simulink model "OMAP"  (R2018b)
settings: Solver=FixedStepDiscrete  StartTime=0.0  StopTime=10.0  FixedStep=0.01  RelTol=1e-3
values from neighbouring files (symbols this model uses):
  Clb_ICADirect_LaneDisp_StateFive = Simulink.Parameter    [omap_ver_442.m]
  Clb_ICADirect_LaneDisp_StateFour = Simulink.Parameter    [omap_ver_442.m]
  Clb_ICADirect_LaneDisp_StateOne = Simulink.Parameter    [omap_ver_442.m]
  Clb_ICADirect_LaneDisp_StateThree = Simulink.Parameter    [omap_ver_442.m]
  Clb_ICADirect_LaneDisp_StateTwo = Simulink.Parameter    [omap_ver_442.m]
  Clb_ICADirect_LaneDisp_StateZero = Simulink.Parameter    [omap_ver_442.m]
  Clb_ICADirect_LaneDispSW = Simulink.Parameter    [omap_ver_442.m]
  Clb_ICADirect_TrnLghtsCom_Switch = Simulink.Parameter    [omap_ver_442.m]
  Clb_ICADirect_TrnLghtsCom_Value = Simulink.Parameter    [omap_ver_442.m]
  Clb_ICADirect_TrnLghtsCrtl_Inhb = Simulink.Parameter    [omap_ver_442.m]
  OMAP_ACCAEB_EMSESC_Decel = Simulink.Parameter    [omap_ver_442.m]
  OMAP_ACCFCW_IC_Decel = Simulink.Parameter    [omap_ver_442.m]
  OMAP_clb_ACC_RVVReqType = Simulink.Parameter    [omap_ver_442.m]
  OMAP_clb_ACC_RVVReqType_Switch = Simulink.Parameter    [omap_ver_442.m]
  OMAP_clb_ACCHeadwayDisplay = Simulink.Parameter    [omap_ver_442.m]
  OMAP_clb_ACCHeadwayDisplay_Switch = Simulink.Parameter    [omap_ver_442.m]
  OMAP_clb_ACCHeadwayIcon = Simulink.Parameter    [omap_ver_442.m]
  OMAP_clb_ACCHeadwayIcon_Switch = Simulink.Parameter    [omap_ver_442.m]
  OMAP_clb_ACCMessagePrompt = Simulink.Parameter    [omap_ver_442.m]
  OMAP_clb_ACCMessagePrompt_Switch = Simulink.Parameter    [omap_ver_442.m]
  OMAP_clb_ACCRequestEPB = Simulink.Parameter    [omap_ver_442.m]
  OMAP_clb_ACCRequestEPB_Switch = Simulink.Parameter    [omap_ver_442.m]
  OMAP_clb_ACCSetSpeed = Simulink.Parameter    [omap_ver_442.m]
  OMAP_clb_ACCSetSpeed_Switch = Simulink.Parameter    [omap_ver_442.m]
  OMAP_clb_ACCSetSpeedDis = Simulink.Parameter    [omap_ver_442.m]
  OMAP_clb_ACCSetSpeedDis_Switch = Simulink.Parameter    [omap_ver_442.m]
  OMAP_clb_ACCState = Simulink.Parameter    [omap_ver_442.m]
  OMAP_clb_ACCState_Switch = Simulink.Parameter    [omap_ver_442.m]
  OMAP_clb_ACCStatusIconDis = Simulink.Parameter    [omap_ver_442.m]
  OMAP_clb_ACCStatusIconDis_Switch = Simulink.Parameter    [omap_ver_442.m]
  OMAP_clb_ACCTorqueReq = Simulink.Parameter    [omap_ver_442.m]
  OMAP_clb_ACCTorqueReq_Switch = Simulink.Parameter    [omap_ver_442.m]
  OMAP_clb_ADAS_State = Simulink.Parameter    [omap_ver_442.m]
  OMAP_clb_ADAS_State_Switch = Simulink.Parameter    [omap_ver_442.m]
  OMAP_clb_AEBAlertReq = Simulink.Parameter    [omap_ver_442.m]
  OMAP_clb_AEBAlertReq_Switch = Simulink.Parameter    [omap_ver_442.m]
  OMAP_clb_AEBBrakingProg = Simulink.Parameter    [omap_ver_442.m]
  OMAP_clb_AEBBrakingProg_Switch = Simulink.Parameter    [omap_ver_442.m]
  OMAP_clb_AEBFaultStatus = Simulink.Parameter    [omap_ver_442.m]
  OMAP_clb_AEBFaultStatus_Switch = Simulink.Parameter    [omap_ver_442.m]
  OMAP_clb_AEBMassageDisp = Simulink.Parameter    [omap_ver_442.m]
  OMAP_clb_AEBMassageDisp_Switch = Simulink.Parameter    [omap_ver_442.m]
  OMAP_clb_AEBState = Simulink.Parameter    [omap_ver_442.m]
  OMAP_clb_AEBState_Switch = Simulink.Parameter    [omap_ver_442.m]
  OMAP_clb_AEBSwitchStatus = Simulink.Parameter    [omap_ver_442.m]
  OMAP_clb_AEBSwitchStatus_Switch = Simulink.Parameter    [omap_ver_442.m]
  OMAP_clb_BrakeRequest = Simulink.Parameter    [omap_ver_442.m]
  OMAP_clb_BrakeRequest_Switch = Simulink.Parameter    [omap_ver_442.m]
  OMAP_clb_DecelerationSet = Simulink.Parameter    [omap_ver_442.m]
  OMAP_clb_DecelerationSet_Switch = Simulink.Parameter    [omap_ver_442.m]
  OMAP_clb_DecelerationType = Simulink.Parameter    [omap_ver_442.m]
  OMAP_clb_DecelerationType_Switch = Simulink.Parameter    [omap_ver_442.m]
  OMAP_clb_DeclControlReq = Simulink.Parameter    [omap_ver_442.m]
  OMAP_clb_DeclControlReq_Switch = Simulink.Parameter    [omap_ver_442.m]
  OMAP_clb_DownorUpGearMinTime = Simulink.Parameter    [omap_ver_442.m]
  OMAP_clb_DownorUpGearMinTime_Switch = Simulink.Parameter    [omap_ver_442.m]
  OMAP_clb_ELKPopupMessage = Simulink.Parameter    [omap_ver_442.m]
  OMAP_clb_ELKPopupMessage_Switch = Simulink.Parameter    [omap_ver_442.m]
  OMAP_clb_ELKSts = Simulink.Parameter    [omap_ver_442.m]
  OMAP_clb_ELKSts_Switch = Simulink.Parameter    [omap_ver_442.m]
  OMAP_clb_ESAFaultSt = Simulink.Parameter    [omap_ver_442.m]
  OMAP_clb_ESAFaultSt_Switch = Simulink.Parameter    [omap_ver_442.m]
  OMAP_clb_ESARequest = Simulink.Parameter    [omap_ver_442.m]
  OMAP_clb_ESARequest_Switch = Simulink.Parameter    [omap_ver_442.m]
  OMAP_clb_ESAState = Simulink.Parameter    [omap_ver_442.m]
  OMAP_clb_ESAState_Switch = Simulink.Parameter    [omap_ver_442.m]
  OMAP_clb_ESATorqueReq = Simulink.Parameter    [omap_ver_442.m]
  OMAP_clb_ESATorqueReq_Switch = Simulink.Parameter    [omap_ver_442.m]
  OMAP_clb_ESCDriveOff = Simulink.Parameter    [omap_ver_442.m]
  OMAP_clb_ESCDriveOff_Switch = Simulink.Parameter    [omap_ver_442.m]
  OMAP_clb_ESCHoldReq = Simulink.Parameter    [omap_ver_442.m]
  OMAP_clb_ESCHoldReq_Switch = Simulink.Parameter    [omap_ver_442.m]
  OMAP_clb_Handsoffwarning = Simulink.Parameter    [omap_ver_442.m]
  OMAP_clb_Handsoffwarning_Switch = Simulink.Parameter    [omap_ver_442.m]
  OMAP_clb_HapticAlarmReq = Simulink.Parameter    [omap_ver_442.m]
  OMAP_clb_HapticAlarmReq_Switch = Simulink.Parameter    [omap_ver_442.m]
  OMAP_clb_HMIPopupMassage = Simulink.Parameter    [omap_ver_442.m]
  OMAP_clb_HMIPopupMassage_Switch = Simulink.Parameter    [omap_ver_442.m]
  OMAP_clb_HWAActionSts = Simulink.Parameter    [omap_ver_442.m]
  OMAP_clb_HWAActionSts_Switch = Simulink.Parameter    [omap_ver_442.m]
  OMAP_clb_HWAMode = Simulink.Parameter    [omap_ver_442.m]
  OMAP_clb_HWAMode_Switch = Simulink.Parameter    [omap_ver_442.m]
  OMAP_clb_HWATurnOnIdctr = Simulink.Parameter    [omap_ver_442.m]
  OMAP_clb_HWATurnOnIdctr_Switch = Simulink.Parameter    [omap_ver_442.m]
  OMAP_clb_ICAMassageDisp = Simulink.Parameter    [omap_ver_442.m]
  OMAP_clb_ICAMassageDisp_Switch = Simulink.Parameter    [omap_ver_442.m]
  OMAP_clb_ICAStatusIcon = Simulink.Parameter    [omap_ver_442.m]
  OMAP_clb_ICAStatusIcon_Switch = Simulink.Parameter    [omap_ver_442.m]
  OMAP_clb_ISLCDriverRemind = Simulink.Parameter    [omap_ver_442.m]
  OMAP_clb_ISLCDriverRemind_Switch = Simulink.Parameter    [omap_ver_442.m]
  OMAP_clb_ISLCState = Simulink.Parameter    [omap_ver_442.m]
  OMAP_clb_ISLCState_Switch = Simulink.Parameter    [omap_ver_442.m]
  OMAP_clb_JAFaultSt = Simulink.Parameter    [omap_ver_442.m]
  OMAP_clb_JAFaultSt_Switch = Simulink.Parameter    [omap_ver_442.m]
  OMAP_clb_LCAPopupMessage = Simulink.Parameter    [omap_ver_442.m]
  OMAP_clb_LCAPopupMessage_Switch = Simulink.Parameter    [omap_ver_442.m]
  OMAP_clb_LCAStatusDisplay = Simulink.Parameter    [omap_ver_442.m]
  OMAP_clb_LCAStatusDisplay_Switch = Simulink.Parameter    [omap_ver_442.m]
  OMAP_clb_LDWStatusDisplay = Simulink.Parameter    [omap_ver_442.m]
  OMAP_clb_LDWStatusDisplay_Switch = Simulink.Parameter    [omap_ver_442.m]
  OMAP_clb_LDWWarningSt = Simulink.Parameter    [omap_ver_442.m]
  OMAP_clb_LDWWarningSt_Switch = Simulink.Parameter    [omap_ver_442.m]
  OMAP_clb_LightControlValid = Simulink.Parameter    [omap_ver_442.m]
  OMAP_clb_LightControlValid_Switch = Simulink.Parameter    [omap_ver_442.m]
  OMAP_clb_LKAActivation = Simulink.Parameter    [omap_ver_442.m]
  OMAP_clb_LKAActivation_Switch = Simulink.Parameter    [omap_ver_442.m]
  OMAP_clb_LKAAngleReq = Simulink.Parameter    [omap_ver_442.m]
  OMAP_clb_LKAAngleReq_Switch = Simulink.Parameter    [omap_ver_442.m]
  OMAP_clb_LKAMode = Simulink.Parameter    [omap_ver_442.m]
  OMAP_clb_LKAMode_Switch = Simulink.Parameter    [omap_ver_442.m]
  OMAP_clb_LKAorELK_CoolTime = Simulink.Parameter    [omap_ver_442.m]
  OMAP_clb_LKAState = Simulink.Parameter    [omap_ver_442.m]
  OMAP_clb_LKAState_Switch = Simulink.Parameter    [omap_ver_442.m]
  OMAP_clb_LKAStatusDisplay = Simulink.Parameter    [omap_ver_442.m]
  OMAP_clb_LKAStatusDisplay_Switch = Simulink.Parameter    [omap_ver_442.m]
  OMAP_clb_LKASwitchState = Simulink.Parameter    [omap_ver_442.m]
  OMAP_clb_LKASwitchState_Switch = Simulink.Parameter    [omap_ver_442.m]
  OMAP_clb_LKATorqFactReq = Simulink.Parameter    [omap_ver_442.m]
  OMAP_clb_LKATorqFactReq_Switch = Simulink.Parameter    [omap_ver_442.m]
  OMAP_clb_PrefillRequest = Simulink.Parameter    [omap_ver_442.m]
  ... (+36 more)
libraries: simulink x184, canmsglib x2
(part 1 of 14)
settings Model: Creator=许阁  LastModifiedBy=许阁
settings OptimizationCC: BlockReduction=off  DefaultParameterBehavior=Inlined  DefaultUnderspecifiedDataType=single  EnhancedBackFolding=on  PassReuseOutputArgsAs=Individual arguments  ZeroExternalMemoryAtStartup=off  ZeroInternalMemoryAtStartup=off  OptimizeBlockOrder=speed  DifferentSizesBufferReuse=on  OptimizationCustomize=off
settings DebuggingCC: ParameterTunabilityLossMsg=error
settings SFSimCC: MATLABDynamicMemAlloc=off
settings RTWCC: SystemTargetFile=autosar.tlc  GenCodeOnly=on  TemplateMakefile=ert_default_tmf  Description=AUTOSAR  GenerateReport=on  IncludeHyperlinkInReport=on  LaunchReport=on  GenerateTraceInfo=on  GenerateTraceReport=on  GenerateTraceReportSl=on  GenerateTraceReportSf=on  GenerateTraceReportEml=on  GenerateCodeMetricsReport=on
settings CodeAppCC: ForceParamTrailComments=on  IgnoreCustomStorageClasses=off  OperatorAnnotations=on  SimulinkDataObjDesc=on  SFDataObjDesc=on  InsertBlockDesc=on
settings STFCustomTargetCC: TargetLangStandard=C99 (ISO)  MultiwordLength=256  ParMdlRefBuildCompliant=on  CompOptLevelCompliant=on  IncludeMdlTerminateFcn=off  CombineOutputUpdateFcns=on  SuppressErrorStatus=on  ERTCustomFileBanners=on  SupportNonFinite=off  SupportComplex=off  SupportContinuousTime=off  SupportNonInlinedSFcns=off  RemoveResetFunc=on  MATLABClassNameForMDSCustomization=Simulink.SoftwareTarget.ERTCustomization  AutosarCompliant=on  UseToolchainInfoCompliant=on  LookupTableObjectStructAxisOrder=2,1,3,4,...  LUTObjectStructOrderEvenSpacing=Size,Table,Breakpoints  SystemTargetFile=autosar.tlc
settings ERTTargetCC: TargetLangStandard=C99 (ISO)  ConcurrentExecutionCompliant=off  IncludeMdlTerminateFcn=off  SuppressErrorStatus=on  SupportNonFinite=off  SupportComplex=off  ModelStepFunctionPrototypeControlCompliant=off  CPPClassGenCompliant=off  AutosarCompliant=on  LookupTableObjectStructAxisOrder=2,1,3,4,...  LUTObjectStructOrderEvenSpacing=Size,Table,Breakpoints  GenerateASAP2=on  InlinedParameterPlacement=NonHierarchical  ERTCustomFileTemplate=example_file_process.tlc

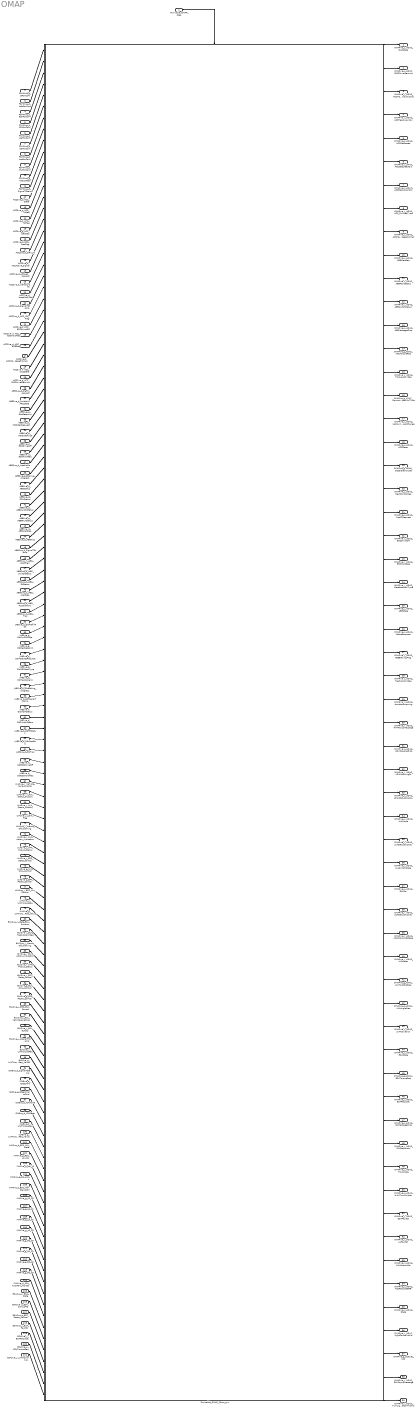
== system OMAP ==
  Runnable_OMAP_Step : Inport  SampleTime=0.01  OutputFunctionCall=on
  FDMMve_d_JaFcnConf : Inport  Port=2  OutDataTypeStr=UInt16  PortDimensions=1
  FDMMve_d_AebFcnConf : Inport  Port=3  OutDataTypeStr=UInt16  PortDimensions=1
  FDMMve_d_EsaFcnConf : Inport  Port=4  OutDataTypeStr=UInt16  PortDimensions=1
  FDMMve_d_ElkFcnConf : Inport  Port=5  OutDataTypeStr=UInt16  PortDimensions=1
  FDMMve_d_LkaFcnConf : Inport  Port=6  OutDataTypeStr=UInt16  PortDimensions=1
  FDMMve_d_IcaFcnConf : Inport  Port=7  OutDataTypeStr=UInt16  PortDimensions=1
  FDMMve_d_AccFcnConf : Inport  Port=8  OutDataTypeStr=UInt16  PortDimensions=1
  FDMMve_d_EwFcnConf : Inport  Port=9  OutDataTypeStr=UInt16  PortDimensions=1
  FDMMve_g_Adas2Fapa : Inport  Port=10  OutDataTypeStr=UInt32  PortDimensions=1
  FDMMve_d_SignalTStamp : Inport  Port=11  OutDataTypeStr=UInt16  PortDimensions=1
  ACCSve_d_ACC_State : Inport  Port=12  OutDataTypeStr=UInt16  PortDimensions=1
  ACCSve_g_ACC_TqReq : Inport  Port=13  OutDataTypeStr=T_M_Nm_Float32  PortDimensions=1
  ACCSve_d_ACC_TqFlag : Inport  Port=14  OutDataTypeStr=UInt16  PortDimensions=1
  ACCSve_g_ACC_DecReq : Inport  Port=15  OutDataTypeStr=T_M_Nm_Float32  PortDimensions=1
  ACCSve_d_ACC_DecFlag : Inport  Port=16  OutDataTypeStr=UInt16  PortDimensions=1
  ACCSve_d_CIPV_ID : Inport  Port=17  OutDataTypeStr=UInt16  PortDimensions=1
  ACCSve_d_ACCActive_Signal : Inport  Port=18  OutDataTypeStr=UInt16  PortDimensions=1
  ACCSve_d_ACC_go_request : Inport  Port=19  OutDataTypeStr=UInt16  PortDimensions=1
  ACCSve_d_VelocitySet : Inport  Port=20  OutDataTypeStr=UInt16  PortDimensions=1
  ACCSve_d_HeadWaySet : Inport  Port=21  OutDataTypeStr=UInt16  PortDimensions=1
  ACCSve_d_SignalTStamp : Inport  Port=22  OutDataTypeStr=UInt16  PortDimensions=1
  ACCSve_d_ACC_ICA_Flag : Inport  Port=23  OutDataTypeStr=UInt16  PortDimensions=1
  ACCSve_d_ACC_ESCDriveOff : Inport  Port=24  OutDataTypeStr=UInt16  PortDimensions=1
  ACCSve_d_ACC_ESCHoldReq : Inport  Port=25  OutDataTypeStr=UInt16  PortDimensions=1
  ACCSve_d_ACC_EPBReq : Inport  Port=26  OutDataTypeStr=UInt16  PortDimensions=1
  ACCSve_d_ACCMessagePrompt : Inport  Port=27  OutDataTypeStr=UInt16
  ACCSve_d_ACC_ISLCState : Inport  Port=28  OutDataTypeStr=UInt16  PortDimensions=1
  ACCSve_d_ACC_ISLCDriverRemind : Inport  Port=29  OutDataTypeStr=UInt16  PortDimensions=1
  AEBSve_d_Prefill_request : Inport  Port=30  OutDataTypeStr=UInt16  PortDimensions=1
  AEBSve_d_functionFARCState : Inport  Port=31  OutDataTypeStr=UInt16  PortDimensions=1
  AEBSve_g_DecSetpoint : Inport  Port=32  OutDataTypeStr=T_M_Nm_Float32  PortDimensions=1
  AEBSve_d_MDDdecRequest : Inport  Port=33  OutDataTypeStr=UInt16  PortDimensions=1
  AEBSve_d_MDDdecType : Inport  Port=34  OutDataTypeStr=UInt16  PortDimensions=1
  AEBSve_d_ESCDriveOff : Inport  Port=35  OutDataTypeStr=UInt16  PortDimensions=1
  AEBSve_d_ESCHoldReq : Inport  Port=36  OutDataTypeStr=UInt16  PortDimensions=1
  AEBSve_d_HapticAlarm : Inport  Port=37  OutDataTypeStr=UInt16  PortDimensions=1
  AEBSve_d_Braking_progress : Inport  Port=38  OutDataTypeStr=UInt16  PortDimensions=1
  AEBSve_d_AEBStatus : Inport  Port=39  OutDataTypeStr=UInt16  PortDimensions=1
  AEBSve_d_FCWStatus : Inport  Port=40  OutDataTypeStr=UInt16  PortDimensions=1
  AEBSve_d_AEBSwitchStatus : Inport  Port=41  OutDataTypeStr=UInt16  PortDimensions=1
  AEBSve_d_AEBFaultStatus : Inport  Port=42  OutDataTypeStr=UInt16  PortDimensions=1
  AEBSve_d_AEBAlertReq : Inport  Port=43  OutDataTypeStr=UInt16  PortDimensions=1
  AEBSve_d_AEBTips : Inport  Port=44  OutDataTypeStr=UInt16  PortDimensions=1
  AEBSve_d_SignalTStamp : Inport  Port=45  OutDataTypeStr=UInt16  PortDimensions=1
  AEBSve_d_JABS_AlertSign : Inport  Port=46  OutDataTypeStr=UInt16  PortDimensions=1
  AEBSve_d_JABS_SwitchStatus : Inport  Port=47  OutDataTypeStr=UInt16  PortDimensions=1
  AEBSve_d_JABS_FltStatus : Inport  Port=48  OutDataTypeStr=UInt16  PortDimensions=1
  AEBSve_d_JABS_AlertReq : Inport  Port=49  OutDataTypeStr=UInt16  PortDimensions=1
  AEBSve_d_JABS_HapticAlarm : Inport  Port=50  OutDataTypeStr=UInt16  PortDimensions=1
  AEBSve_d_JABS_Tips : Inport  Port=51  OutDataTypeStr=UInt16  PortDimensions=1
  JABSve_d_DbPrefillReq : Inport  Port=52  OutDataTypeStr=UInt16  PortDimensions=1
  JABSve_d_DbFunFARCSta : Inport  Port=53  OutDataTypeStr=UInt16  PortDimensions=1
  JABSve_g_DbDecSetpoint : Inport  Port=54  OutDataTypeStr=T_M_Nm_Float32  PortDimensions=1
  JABSve_d_DbMDDdecRequest : Inport  Port=55  OutDataTypeStr=UInt16  PortDimensions=1
  JABSve_d_DbMDDdecType : Inport  Port=56  OutDataTypeStr=UInt16  PortDimensions=1
  JABSve_d_DbHapticAlarm : Inport  Port=57  OutDataTypeStr=UInt16  PortDimensions=1
  JABSve_d_DbBraking_progress : Inport  Port=58  OutDataTypeStr=UInt16  PortDimensions=1
  JABSve_d_DbSignalTStamp : Inport  Port=59  OutDataTypeStr=UInt16  PortDimensions=1
  JABSve_d_DbJACWStatus : Inport  Port=60  OutDataTypeStr=UInt16  PortDimensions=1
  JABSve_d_DbSwitchStatus : Inport  Port=61  OutDataTypeStr=UInt16  PortDimensions=1
  JABSve_d_DbFltStatus : Inport  Port=62  OutDataTypeStr=UInt16  PortDimensions=1
  JABSve_d_DbAlertReq : Inport  Port=63  OutDataTypeStr=UInt16  PortDimensions=1
  JABSve_d_DbTips : Inport  Port=64  OutDataTypeStr=UInt16  PortDimensions=1
  JABSve_d_DbESCDriveOff : Inport  Port=65  OutDataTypeStr=UInt16  PortDimensions=1
  JABSve_d_DbESCHoldReq : Inport  Port=66  OutDataTypeStr=UInt16  PortDimensions=1
  LKASve_y_Vehicle_Lane_Display : Inport  Port=67  OutDataTypeStr=UInt8  PortDimensions=1
  LKASve_y_LDW_Status_Display : Inport  Port=68  OutDataTypeStr=UInt8  PortDimensions=1
  LKASve_y_LKA_Status_Display : Inport  Port=69  OutDataTypeStr=UInt8  PortDimensions=1
  LKASve_y_LDW_Flag : Inport  Port=70  OutDataTypeStr=UInt8  PortDimensions=1
  LKASve_y_Hands_Off_Warning : Inport  Port=71  OutDataTypeStr=UInt8  PortDimensions=1
  LKASve_y_LKA_Action_Indication : Inport  Port=72  OutDataTypeStr=UInt8  PortDimensions=1
  LKASve_y_HMI_Popup_Status : Inport  Port=73  OutDataTypeStr=UInt8  PortDimensions=1
  LKASve_y_EPS_State_Control : Inport  Port=74  OutDataTypeStr=UInt8  PortDimensions=1
  LKASve_g_LKA_SWA_Control : Inport  Port=75  OutDataTypeStr=T_M_Nm_Float32  PortDimensions=1
  LKASve_g_EPS_Factor_Control : Inport  Port=76  OutDataTypeStr=T_M_Nm_Float32  PortDimensions=1
  LKASve_y_EPS_LKA_Control : Inport  Port=77  OutDataTypeStr=UInt8  PortDimensions=1
  LKASve_y_LKATorqueReq : Inport  Port=78  OutDataTypeStr=UInt8  PortDimensions=1
  LKASve_g_LKATorqueReq_Value : Inport  Port=79  OutDataTypeStr=T_M_Nm_Float32  PortDimensions=1
  ELKSve_y_state_ELK_function : Inport  Port=80  OutDataTypeStr=UInt8  PortDimensions=1
  ELKSve_y_ELK_HapticAlarmReq : Inport  Port=81  OutDataTypeStr=UInt8  PortDimensions=1
  ELKSve_y_Hands_Off_Warning : Inport  Port=82  OutDataTypeStr=UInt8  PortDimensions=1
  ELKSve_y_ELK_Action_Indication : Inport  Port=83  OutDataTypeStr=UInt8  PortDimensions=1
  ELKSve_y_HMI_Popup_Status : Inport  Port=84  OutDataTypeStr=UInt8  PortDimensions=1
  ELKSve_y_EPS_State_Control : Inport  Port=85  OutDataTypeStr=UInt8  PortDimensions=1
  ELKSve_g_ELK_SWA_Control : Inport  Port=86  OutDataTypeStr=T_M_Nm_Float32  PortDimensions=1
  ELKSve_g_EPS_Factor_Control : Inport  Port=87  OutDataTypeStr=T_M_Nm_Float32  PortDimensions=1
  ELKSve_y_EPS_ELK_Control : Inport  Port=88  OutDataTypeStr=UInt8  PortDimensions=1
  ELKSve_y_ELK_VehicleLaneDisp : Inport  Port=89  OutDataTypeStr=UInt8  PortDimensions=1
  ELKSve_y_ELK_ELKSts : Inport  Port=90  OutDataTypeStr=UInt8  PortDimensions=1
  ELKSve_y_SignalTStamp : Inport  Port=91  OutDataTypeStr=UInt8  PortDimensions=1
  ELKSve_y_LKATorqueReq : Inport  Port=92  OutDataTypeStr=UInt8  PortDimensions=1
  ELKSve_g_LKATorqueReq_Value : Inport  Port=93  OutDataTypeStr=T_M_Nm_Float32  PortDimensions=1
  ICABve_d_SignalTStamp : Inport  Port=94  OutDataTypeStr=UInt16  PortDimensions=1
  ICABva_d_ICAB2HMI : Inport  Port=95  OutDataTypeStr=UInt16  PortDimensions=20
  ICABve_g_SteerAngleCmd : Inport  Port=96  OutDataTypeStr=T_M_Nm_Float32  PortDimensions=1
  ICABve_d_ICAMode : Inport  Port=97  OutDataTypeStr=UInt16  PortDimensions=1
  ICABve_d_ICAState : Inport  Port=98  OutDataTypeStr=UInt16  PortDimensions=1
  ICABve_d_LKATorqueReq : Inport  Port=99  OutDataTypeStr=UInt16  PortDimensions=1
  ICABve_g_LKATorqueReq_Value : Inport  Port=100  OutDataTypeStr=T_M_Nm_Float32  PortDimensions=1
  IMAPve_d_EPS_LKA_State : Inport  Port=101  OutDataTypeStr=UInt16  PortDimensions=1
  IMAPve_g_ESC_LonAcc : Inport  Port=102  OutDataTypeStr=T_M_Nm_Float32  PortDimensions=1
  IMAPva_d_obj_id : Inport  Port=103  OutDataTypeStr=UInt16  PortDimensions=40
  IMAPva_g_obj_pos_x : Inport  Port=104  OutDataTypeStr=T_M_Nm_Float32  PortDimensions=40
  IMAPve_d_ESC_Veh_Standstill : Inport  Port=105  OutDataTypeStr=UInt16  PortDimensions=1
  IMAPve_g_L0_C0 : Inport  Port=106  OutDataTypeStr=T_M_Nm_Float32  PortDimensions=1
  IMAPve_g_L0_C1 : Inport  Port=107  OutDataTypeStr=T_M_Nm_Float32  PortDimensions=1
  IMAPve_g_L0_C2 : Inport  Port=108  OutDataTypeStr=T_M_Nm_Float32  PortDimensions=1
  IMAPve_g_L0_C3 : Inport  Port=109  OutDataTypeStr=T_M_Nm_Float32  PortDimensions=1
  IMAPve_g_R0_C0 : Inport  Port=110  OutDataTypeStr=T_M_Nm_Float32  PortDimensions=1
  IMAPve_g_R0_C1 : Inport  Port=111  OutDataTypeStr=T_M_Nm_Float32  PortDimensions=1
  IMAPve_g_R0_C2 : Inport  Port=112  OutDataTypeStr=T_M_Nm_Float32  PortDimensions=1
  IMAPve_g_R0_C3 : Inport  Port=113  OutDataTypeStr=T_M_Nm_Float32  PortDimensions=1
  IMAPve_d_APA_AutoPark_WorkSt : Inport  Port=114  OutDataTypeStr=UInt16  PortDimensions=1
  ESASve_y_ESA_State : Inport  Port=115  OutDataTypeStr=UInt8
  ESASve_g_ESA_SWA_CMD : Inport  Port=116  OutDataTypeStr=T_M_Nm_Float32
  ESASve_g_EPS_Factor_Control : Inport  Port=117  OutDataTypeStr=T_M_Nm_Float32
  ESASve_y_ESA_FaultSt : Inport  Port=118  OutDataTypeStr=UInt8
  ESASve_y_ESARequest : Inport  Port=119  OutDataTypeStr=UInt8
  ESASve_y_ESATorqueReq : Inport  Port=120  OutDataTypeStr=T_M_Nm_Float32
  ESASve_y_LKAActivation : Inport  Port=121  OutDataTypeStr=UInt8
  Runnable_OMAP_10ms_sys : Subsystem
  OMAPve_y_ADAS_ISLCState : Outport  OutDataTypeStr=UInt8  PortDimensions=1
  OMAPve_y_ADAS_ISLCDriverRemind : Outport  Port=2  OutDataTypeStr=UInt8  PortDimensions=1
  OMAPve_y_ADAS_ACCHeadwayDisplay : Outport  Port=3  OutDataTypeStr=UInt8  PortDimensions=1
  OMAPve_y_ADAS_ACCHeadwayIcon : Outport  Port=4  OutDataTypeStr=UInt8  PortDimensions=1
  OMAPve_y_ADAS_ACCSetSpeed : Outport  Port=5  OutDataTypeStr=UInt8  PortDimensions=1
  OMAPve_y_ADAS_ACCSetSpeedDis : Outport  Port=6  OutDataTypeStr=UInt8  PortDimensions=1
  OMAPve_y_ADAS_ACCStatusIconDis : Outport  Port=7  OutDataTypeStr=UInt8  PortDimensions=1
  OMAPve_y_ADAS_ACC_RVVReqType : Outport  Port=8  OutDataTypeStr=UInt8  PortDimensions=1
  OMAPve_y_ADAS_ACCMessagePrompt : Outport  Port=9  OutDataTypeStr=UInt8  PortDimensions=1
  OMAPve_y_ADAS_AEBAlertReq : Outport  Port=10  OutDataTypeStr=UInt8  PortDimensions=1
  OMAPve_y_ADAS_AEBFaultStatus : Outport  Port=11  OutDataTypeStr=UInt8  PortDimensions=1
  OMAPve_y_ADAS_AEBSwitchStatus : Outport  Port=12  OutDataTypeStr=UInt8  PortDimensions=1
  OMAPve_y_ADAS_AEBMassageDisp : Outport  Port=13  OutDataTypeStr=UInt8  PortDimensions=1
  OMAPve_g_ADAS_ACCTorqueReq : Outport  Port=14  OutDataTypeStr=T_M_Nm_Float32  PortDimensions=1
  OMAPve_y_ADAS_TorqueActivReq : Outport  Port=15  OutDataTypeStr=UInt8  PortDimensions=1
  OMAPve_g_ADAS_DownorUpGearMinTime : Outport  Port=16  OutDataTypeStr=T_M_Nm_Float32  PortDimensions=1
  OMAPve_y_ADAS_UpDownGearChange : Outport  Port=17  OutDataTypeStr=UInt8  PortDimensions=1
  OMAPve_y_ADAS_ACCState : Outport  Port=18  OutDataTypeStr=UInt8  PortDimensions=1
  OMAPve_g_ADAS_DecelerationSet : Outport  Port=19  OutDataTypeStr=T_M_Nm_Float32  PortDimensions=1
  OMAPve_y_ADAS_DeclControlReq : Outport  Port=20  OutDataTypeStr=UInt8  PortDimensions=1
  OMAPve_y_ADAS_PrefillRequest : Outport  Port=21  OutDataTypeStr=UInt8  PortDimensions=1
  OMAPve_y_ADAS_ESCDriveOff : Outport  Port=22  OutDataTypeStr=UInt8  PortDimensions=1
  OMAPve_y_ADAS_ESCHoldReq : Outport  Port=23  OutDataTypeStr=UInt8  PortDimensions=1
  OMAPve_y_ADAS_DecelerationType : Outport  Port=24  OutDataTypeStr=UInt8  PortDimensions=1
  OMAPve_y_ADAS_AEBState : Outport  Port=25  OutDataTypeStr=UInt8  PortDimensions=1
  OMAPve_y_ADAS_BrakeRequest : Outport  Port=26  OutDataTypeStr=UInt8  PortDimensions=1
  OMAPve_y_ADAS_AEBBrakingProg : Outport  Port=27  OutDataTypeStr=UInt8  PortDimensions=1
  OMAPve_y_ADAS_HapticAlarmReq : Outport  Port=28  OutDataTypeStr=UInt8  PortDimensions=1
  OMAPve_y_ADAS_Handsoffwarning : Outport  Port=29  OutDataTypeStr=UInt8  PortDimensions=1
  OMAPve_y_ADAS_HMIPopupMassage : Outport  Port=30  OutDataTypeStr=UInt8  PortDimensions=1
  OMAPve_y_ADAS_VehicleLaneDisp : Outport  Port=31  OutDataTypeStr=UInt8  PortDimensions=1
  OMAPve_y_ADAS_LDWWarningSt : Outport  Port=32  OutDataTypeStr=UInt8  PortDimensions=1
  OMAPve_y_ADAS_LDWStatusDisplay : Outport  Port=33  OutDataTypeStr=UInt8  PortDimensions=1
  OMAPve_y_ADAS_LKAMode : Outport  Port=34  OutDataTypeStr=UInt8  PortDimensions=1
  OMAPve_y_ADAS_LKAStatusDisplay : Outport  Port=35  OutDataTypeStr=UInt8  PortDimensions=1
  OMAPve_y_ADAS_LKASwitchState : Outport  Port=36  OutDataTypeStr=UInt8  PortDimensions=1
  OMAPve_y_ADAS_ELKSts : Outport  Port=37  OutDataTypeStr=UInt8  PortDimensions=1
  OMAPve_y_ADAS_LCAStatusDisplay : Outport  Port=38  OutDataTypeStr=UInt8  PortDimensions=1
  OMAPve_y_ADAS_LCAPopupMessage : Outport  Port=39  OutDataTypeStr=UInt8  PortDimensions=1
  OMAPve_y_ADAS_LKAState : Outport  Port=40  OutDataTypeStr=UInt8  PortDimensions=1
  OMAPve_g_ADAS_LKATorqFactReq : Outport  Port=41  OutDataTypeStr=T_M_Nm_Float32  PortDimensions=1
  OMAPve_g_ADAS_LKAAngleReq : Outport  Port=42  OutDataTypeStr=T_M_Nm_Float32  PortDimensions=1
  OMAPve_y_ADAS_LKAActivation : Outport  Port=43  OutDataTypeStr=UInt8  PortDimensions=1
  OMAPve_y_ADAS_ESAState : Outport  Port=44  OutDataTypeStr=UInt8  PortDimensions=1
  OMAPve_g_ADAS_ESATorqueReq : Outport  Port=45  OutDataTypeStr=T_M_Nm_Float32  PortDimensions=1
  OMAPve_y_ADAS_ESARequest : Outport  Port=46  OutDataTypeStr=UInt8  PortDimensions=1
  OMAPve_y_ADAS_ICAMassageDisp : Outport  Port=47  OutDataTypeStr=UInt8  PortDimensions=1
  OMAPve_y_ADAS_ICAStatusIcon : Outport  Port=48  OutDataTypeStr=UInt8  PortDimensions=1
  OMAPve_y_ADAS_HWAMode : Outport  Port=49  OutDataTypeStr=UInt8  PortDimensions=1
  OMAPve_y_ADAS_HWATurnOnIdctr : Outport  Port=50  OutDataTypeStr=UInt8  PortDimensions=1
  OMAPve_y_ADAS_ESAFaultSt : Outport  Port=51  OutDataTypeStr=UInt8  PortDimensions=1
  OMAPve_y_ADAS_JAFaultSt : Outport  Port=52  OutDataTypeStr=UInt8  PortDimensions=1
  OMAPve_y_ADAS_HWAActionSts : Outport  Port=53  OutDataTypeStr=UInt8  PortDimensions=1
  OMAPve_y_ADAS_ACCRequestEPB : Outport  Port=54  OutDataTypeStr=UInt8  PortDimensions=1
  OMAPve_y_ADAS_State : Outport  Port=55  OutDataTypeStr=UInt8  PortDimensions=1
  OMAPve_y_ADAS_LightControlValid : Outport  Port=56  OutDataTypeStr=UInt8  PortDimensions=1
  OMAPve_g_ob019L_100 : Outport  Port=57  OutDataTypeStr=UInt32  PortDimensions=1
  OMAPve_y_ADAS_ELKPopupMessage : Outport  Port=58  OutDataTypeStr=UInt8
  OMAPve_y_ADAS_TurnLightsCommand : Outport  Port=59  OutDataTypeStr=UInt8
  wires:
  Runnable_OMAP_Step/1 -> Runnable_OMAP_10ms_sys/Trigger
  IMAPve_d_EPS_LKA_State/1 -> Runnable_OMAP_10ms_sys/100(IMAPve_d_EPS_LKA_State)
  ELKSve_g_EPS_Factor_Control/1 -> Runnable_OMAP_10ms_sys/86(ELKSve_g_EPS_Factor_Control)
  ELKSve_y_ELK_ELKSts/1 -> Runnable_OMAP_10ms_sys/89(ELKSve_y_ELK_ELKSts)
  ELKSve_y_HMI_Popup_Status/1 -> Runnable_OMAP_10ms_sys/83(ELKSve_y_HMI_Popup_Status)
  ELKSve_y_ELK_HapticAlarmReq/1 -> Runnable_OMAP_10ms_sys/80(ELKSve_y_ELK_HapticAlarmReq)
  LKASve_g_EPS_Factor_Control/1 -> Runnable_OMAP_10ms_sys/75(LKASve_g_EPS_Factor_Control)
  LKASve_y_EPS_LKA_Control/1 -> Runnable_OMAP_10ms_sys/76(LKASve_y_EPS_LKA_Control)
  LKASve_y_HMI_Popup_Status/1 -> Runnable_OMAP_10ms_sys/72(LKASve_y_HMI_Popup_Status)
  LKASve_y_LKA_Status_Display/1 -> Runnable_OMAP_10ms_sys/68(LKASve_y_LKA_Status_Display)
  LKASve_y_LDW_Flag/1 -> Runnable_OMAP_10ms_sys/69(LKASve_y_LDW_Flag)
  JABSve_d_DbESCHoldReq/1 -> Runnable_OMAP_10ms_sys/65(JABSve_d_DbESCHoldReq)
  LKASve_y_Vehicle_Lane_Display/1 -> Runnable_OMAP_10ms_sys/66(LKASve_y_Vehicle_Lane_Display)
  LKASve_y_Hands_Off_Warning/1 -> Runnable_OMAP_10ms_sys/70(LKASve_y_Hands_Off_Warning)
  LKASve_y_LDW_Status_Display/1 -> Runnable_OMAP_10ms_sys/67(LKASve_y_LDW_Status_Display)
  JABSve_d_DbJACWStatus/1 -> Runnable_OMAP_10ms_sys/59(JABSve_d_DbJACWStatus)
  JABSve_d_DbSwitchStatus/1 -> Runnable_OMAP_10ms_sys/60(JABSve_d_DbSwitchStatus)
  JABSve_d_DbAlertReq/1 -> Runnable_OMAP_10ms_sys/62(JABSve_d_DbAlertReq)
  JABSve_d_DbFltStatus/1 -> Runnable_OMAP_10ms_sys/61(JABSve_d_DbFltStatus)
  JABSve_d_DbBraking_progress/1 -> Runnable_OMAP_10ms_sys/57(JABSve_d_DbBraking_progress)
  JABSve_g_DbDecSetpoint/1 -> Runnable_OMAP_10ms_sys/53(JABSve_g_DbDecSetpoint)
  ELKSve_y_EPS_State_Control/1 -> Runnable_OMAP_10ms_sys/84(ELKSve_y_EPS_State_Control)
  JABSve_d_DbSignalTStamp/1 -> Runnable_OMAP_10ms_sys/58(JABSve_d_DbSignalTStamp)
  JABSve_d_DbESCDriveOff/1 -> Runnable_OMAP_10ms_sys/64(JABSve_d_DbESCDriveOff)
  JABSve_d_DbHapticAlarm/1 -> Runnable_OMAP_10ms_sys/56(JABSve_d_DbHapticAlarm)
  JABSve_d_DbMDDdecRequest/1 -> Runnable_OMAP_10ms_sys/54(JABSve_d_DbMDDdecRequest)
  JABSve_d_DbMDDdecType/1 -> Runnable_OMAP_10ms_sys/55(JABSve_d_DbMDDdecType)
  JABSve_d_DbPrefillReq/1 -> Runnable_OMAP_10ms_sys/51(JABSve_d_DbPrefillReq)
  AEBSve_d_JABS_Tips/1 -> Runnable_OMAP_10ms_sys/50(AEBSve_d_JABS_Tips)
  JABSve_d_DbFunFARCSta/1 -> Runnable_OMAP_10ms_sys/52(JABSve_d_DbFunFARCSta)
  AEBSve_d_JABS_AlertSign/1 -> Runnable_OMAP_10ms_sys/45(AEBSve_d_JABS_AlertSign)
  AEBSve_d_SignalTStamp/1 -> Runnable_OMAP_10ms_sys/44(AEBSve_d_SignalTStamp)
  AEBSve_d_AEBAlertReq/1 -> Runnable_OMAP_10ms_sys/42(AEBSve_d_AEBAlertReq)
  AEBSve_d_JABS_SwitchStatus/1 -> Runnable_OMAP_10ms_sys/46(AEBSve_d_JABS_SwitchStatus)
  ELKSve_g_ELK_SWA_Control/1 -> Runnable_OMAP_10ms_sys/85(ELKSve_g_ELK_SWA_Control)
  IMAPve_g_ESC_LonAcc/1 -> Runnable_OMAP_10ms_sys/101(IMAPve_g_ESC_LonAcc)
  AEBSve_d_AEBSwitchStatus/1 -> Runnable_OMAP_10ms_sys/40(AEBSve_d_AEBSwitchStatus)
  AEBSve_d_HapticAlarm/1 -> Runnable_OMAP_10ms_sys/36(AEBSve_d_HapticAlarm)
  AEBSve_d_FCWStatus/1 -> Runnable_OMAP_10ms_sys/39(AEBSve_d_FCWStatus)
  AEBSve_d_AEBStatus/1 -> Runnable_OMAP_10ms_sys/38(AEBSve_d_AEBStatus)
  AEBSve_d_Braking_progress/1 -> Runnable_OMAP_10ms_sys/37(AEBSve_d_Braking_progress)
  AEBSve_d_AEBFaultStatus/1 -> Runnable_OMAP_10ms_sys/41(AEBSve_d_AEBFaultStatus)
  AEBSve_d_ESCHoldReq/1 -> Runnable_OMAP_10ms_sys/35(AEBSve_d_ESCHoldReq)
  AEBSve_d_MDDdecType/1 -> Runnable_OMAP_10ms_sys/33(AEBSve_d_MDDdecType)
  AEBSve_d_MDDdecRequest/1 -> Runnable_OMAP_10ms_sys/32(AEBSve_d_MDDdecRequest)
  AEBSve_d_functionFARCState/1 -> Runnable_OMAP_10ms_sys/30(AEBSve_d_functionFARCState)
  ACCSve_d_ACC_ESCHoldReq/1 -> Runnable_OMAP_10ms_sys/24(ACCSve_d_ACC_ESCHoldReq)
  AEBSve_g_DecSetpoint/1 -> Runnable_OMAP_10ms_sys/31(AEBSve_g_DecSetpoint)
  ACCSve_d_ACC_ICA_Flag/1 -> Runnable_OMAP_10ms_sys/22(ACCSve_d_ACC_ICA_Flag)
  ACCSve_d_VelocitySet/1 -> Runnable_OMAP_10ms_sys/19(ACCSve_d_VelocitySet)
  ACCSve_d_SignalTStamp/1 -> Runnable_OMAP_10ms_sys/21(ACCSve_d_SignalTStamp)
  ACCSve_d_ACC_TqFlag/1 -> Runnable_OMAP_10ms_sys/13(ACCSve_d_ACC_TqFlag)
  ICABve_d_SignalTStamp/1 -> Runnable_OMAP_10ms_sys/93(ICABve_d_SignalTStamp)
  ACCSve_g_ACC_DecReq/1 -> Runnable_OMAP_10ms_sys/14(ACCSve_g_ACC_DecReq)
  ACCSve_d_CIPV_ID/1 -> Runnable_OMAP_10ms_sys/16(ACCSve_d_CIPV_ID)
  ACCSve_d_ACC_DecFlag/1 -> Runnable_OMAP_10ms_sys/15(ACCSve_d_ACC_DecFlag)
  ACCSve_d_ACC_State/1 -> Runnable_OMAP_10ms_sys/11(ACCSve_d_ACC_State)
  ACCSve_d_ACC_EPBReq/1 -> Runnable_OMAP_10ms_sys/25(ACCSve_d_ACC_EPBReq)
  FDMMve_d_SignalTStamp/1 -> Runnable_OMAP_10ms_sys/10(FDMMve_d_SignalTStamp)
  FDMMve_d_EwFcnConf/1 -> Runnable_OMAP_10ms_sys/8(FDMMve_d_EwFcnConf)
  FDMMve_d_IcaFcnConf/1 -> Runnable_OMAP_10ms_sys/6(FDMMve_d_IcaFcnConf)
  FDMMve_d_LkaFcnConf/1 -> Runnable_OMAP_10ms_sys/5(FDMMve_d_LkaFcnConf)
  AEBSve_d_JABS_HapticAlarm/1 -> Runnable_OMAP_10ms_sys/49(AEBSve_d_JABS_HapticAlarm)
  LKASve_y_LKA_Action_Indication/1 -> Runnable_OMAP_10ms_sys/71(LKASve_y_LKA_Action_Indication)
  FDMMve_d_AccFcnConf/1 -> Runnable_OMAP_10ms_sys/7(FDMMve_d_AccFcnConf)
  FDMMve_d_ElkFcnConf/1 -> Runnable_OMAP_10ms_sys/4(FDMMve_d_ElkFcnConf)
  LKASve_g_LKA_SWA_Control/1 -> Runnable_OMAP_10ms_sys/74(LKASve_g_LKA_SWA_Control)
  FDMMve_d_AebFcnConf/1 -> Runnable_OMAP_10ms_sys/2(FDMMve_d_AebFcnConf)
  FDMMve_d_EsaFcnConf/1 -> Runnable_OMAP_10ms_sys/3(FDMMve_d_EsaFcnConf)
  JABSve_d_DbTips/1 -> Runnable_OMAP_10ms_sys/63(JABSve_d_DbTips)
  AEBSve_d_Prefill_request/1 -> Runnable_OMAP_10ms_sys/29(AEBSve_d_Prefill_request)
  Runnable_OMAP_10ms_sys/1(OMAPve_y_ADAS_ISLCState) -> OMAPve_y_ADAS_ISLCState/1
  IMAPve_g_R0_C3/1 -> Runnable_OMAP_10ms_sys/112(IMAPve_g_R0_C3)
  IMAPve_g_R0_C2/1 -> Runnable_OMAP_10ms_sys/111(IMAPve_g_R0_C2)
  IMAPve_g_L0_C3/1 -> Runnable_OMAP_10ms_sys/108(IMAPve_g_L0_C3)
  IMAPve_g_R0_C1/1 -> Runnable_OMAP_10ms_sys/110(IMAPve_g_R0_C1)
  ACCSve_d_ACCActive_Signal/1 -> Runnable_OMAP_10ms_sys/17(ACCSve_d_ACCActive_Signal)
  IMAPve_g_L0_C2/1 -> Runnable_OMAP_10ms_sys/107(IMAPve_g_L0_C2)
  IMAPve_g_L0_C1/1 -> Runnable_OMAP_10ms_sys/106(IMAPve_g_L0_C1)
  IMAPva_g_obj_pos_x/1 -> Runnable_OMAP_10ms_sys/103(IMAPva_g_obj_pos_x)
  IMAPva_d_obj_id/1 -> Runnable_OMAP_10ms_sys/102(IMAPva_d_obj_id)
  IMAPve_g_L0_C0/1 -> Runnable_OMAP_10ms_sys/105(IMAPve_g_L0_C0)
  ELKSve_y_EPS_ELK_Control/1 -> Runnable_OMAP_10ms_sys/87(ELKSve_y_EPS_ELK_Control)
  ACCSve_d_ACC_ESCDriveOff/1 -> Runnable_OMAP_10ms_sys/23(ACCSve_d_ACC_ESCDriveOff)
  AEBSve_d_ESCDriveOff/1 -> Runnable_OMAP_10ms_sys/34(AEBSve_d_ESCDriveOff)
  ACCSve_d_HeadWaySet/1 -> Runnable_OMAP_10ms_sys/20(ACCSve_d_HeadWaySet)
  IMAPve_d_ESC_Veh_Standstill/1 -> Runnable_OMAP_10ms_sys/104(IMAPve_d_ESC_Veh_Standstill)
  FDMMve_g_Adas2Fapa/1 -> Runnable_OMAP_10ms_sys/9(FDMMve_g_Adas2Fapa)
  Runnable_OMAP_10ms_sys/56(OMAPve_y_ADAS_LightControlValid) -> OMAPve_y_ADAS_LightControlValid/1
  Runnable_OMAP_10ms_sys/55(OMAPve_y_ADAS_State) -> OMAPve_y_ADAS_State/1
  Runnable_OMAP_10ms_sys/54(OMAPve_y_ADAS_ACCRequestEPB) -> OMAPve_y_ADAS_ACCRequestEPB/1
  Runnable_OMAP_10ms_sys/53(OMAPve_y_ADAS_HWAActionSts) -> OMAPve_y_ADAS_HWAActionSts/1
  Runnable_OMAP_10ms_sys/52(OMAPve_y_ADAS_JAFaultSt) -> OMAPve_y_ADAS_JAFaultSt/1
  Runnable_OMAP_10ms_sys/49(OMAPve_y_ADAS_HWAMode) -> OMAPve_y_ADAS_HWAMode/1
  Runnable_OMAP_10ms_sys/48(OMAPve_y_ADAS_ICAStatusIcon) -> OMAPve_y_ADAS_ICAStatusIcon/1
  Runnable_OMAP_10ms_sys/40(OMAPve_y_ADAS_LKAState) -> OMAPve_y_ADAS_LKAState/1
  Runnable_OMAP_10ms_sys/38(OMAPve_y_ADAS_LCAStatusDisplay) -> OMAPve_y_ADAS_LCAStatusDisplay/1
  Runnable_OMAP_10ms_sys/33(OMAPve_y_ADAS_LDWStatusDisplay) -> OMAPve_y_ADAS_LDWStatusDisplay/1
  Runnable_OMAP_10ms_sys/35(OMAPve_y_ADAS_LKAStatusDisplay) -> OMAPve_y_ADAS_LKAStatusDisplay/1
  Runnable_OMAP_10ms_sys/34(OMAPve_y_ADAS_LKAMode) -> OMAPve_y_ADAS_LKAMode/1
  Runnable_OMAP_10ms_sys/36(OMAPve_y_ADAS_LKASwitchState) -> OMAPve_y_ADAS_LKASwitchState/1
  Runnable_OMAP_10ms_sys/29(OMAPve_y_ADAS_Handsoffwarning) -> OMAPve_y_ADAS_Handsoffwarning/1
  ELKSve_y_state_ELK_function/1 -> Runnable_OMAP_10ms_sys/79(ELKSve_y_state_ELK_function)
  Runnable_OMAP_10ms_sys/47(OMAPve_y_ADAS_ICAMassageDisp) -> OMAPve_y_ADAS_ICAMassageDisp/1
  Runnable_OMAP_10ms_sys/32(OMAPve_y_ADAS_LDWWarningSt) -> OMAPve_y_ADAS_LDWWarningSt/1
  FDMMve_d_JaFcnConf/1 -> Runnable_OMAP_10ms_sys/1(FDMMve_d_JaFcnConf)
  ELKSve_y_SignalTStamp/1 -> Runnable_OMAP_10ms_sys/90(ELKSve_y_SignalTStamp)
  Runnable_OMAP_10ms_sys/31(OMAPve_y_ADAS_VehicleLaneDisp) -> OMAPve_y_ADAS_VehicleLaneDisp/1
  Runnable_OMAP_10ms_sys/30(OMAPve_y_ADAS_HMIPopupMassage) -> OMAPve_y_ADAS_HMIPopupMassage/1
  Runnable_OMAP_10ms_sys/27(OMAPve_y_ADAS_AEBBrakingProg) -> OMAPve_y_ADAS_AEBBrakingProg/1
  Runnable_OMAP_10ms_sys/43(OMAPve_y_ADAS_LKAActivation) -> OMAPve_y_ADAS_LKAActivation/1
  Runnable_OMAP_10ms_sys/25(OMAPve_y_ADAS_AEBState) -> OMAPve_y_ADAS_AEBState/1
  Runnable_OMAP_10ms_sys/23(OMAPve_y_ADAS_ESCHoldReq) -> OMAPve_y_ADAS_ESCHoldReq/1
  ELKSve_y_ELK_VehicleLaneDisp/1 -> Runnable_OMAP_10ms_sys/88(ELKSve_y_ELK_VehicleLaneDisp)
  Runnable_OMAP_10ms_sys/42(OMAPve_g_ADAS_LKAAngleReq) -> OMAPve_g_ADAS_LKAAngleReq/1
  Runnable_OMAP_10ms_sys/26(OMAPve_y_ADAS_BrakeRequest) -> OMAPve_y_ADAS_BrakeRequest/1
  Runnable_OMAP_10ms_sys/44(OMAPve_y_ADAS_ESAState) -> OMAPve_y_ADAS_ESAState/1
  Runnable_OMAP_10ms_sys/19(OMAPve_g_ADAS_DecelerationSet) -> OMAPve_g_ADAS_DecelerationSet/1
  AEBSve_d_AEBTips/1 -> Runnable_OMAP_10ms_sys/43(AEBSve_d_AEBTips)
  Runnable_OMAP_10ms_sys/21(OMAPve_y_ADAS_PrefillRequest) -> OMAPve_y_ADAS_PrefillRequest/1
  Runnable_OMAP_10ms_sys/18(OMAPve_y_ADAS_ACCState) -> OMAPve_y_ADAS_ACCState/1
  Runnable_OMAP_10ms_sys/22(OMAPve_y_ADAS_ESCDriveOff) -> OMAPve_y_ADAS_ESCDriveOff/1
  Runnable_OMAP_10ms_sys/39(OMAPve_y_ADAS_LCAPopupMessage) -> OMAPve_y_ADAS_LCAPopupMessage/1
  ICABva_d_ICAB2HMI/1 -> Runnable_OMAP_10ms_sys/94(ICABva_d_ICAB2HMI)
  Runnable_OMAP_10ms_sys/15(OMAPve_y_ADAS_TorqueActivReq) -> OMAPve_y_ADAS_TorqueActivReq/1
  Runnable_OMAP_10ms_sys/41(OMAPve_g_ADAS_LKATorqFactReq) -> OMAPve_g_ADAS_LKATorqFactReq/1
  ACCSve_g_ACC_TqReq/1 -> Runnable_OMAP_10ms_sys/12(ACCSve_g_ACC_TqReq)
  Runnable_OMAP_10ms_sys/28(OMAPve_y_ADAS_HapticAlarmReq) -> OMAPve_y_ADAS_HapticAlarmReq/1
  Runnable_OMAP_10ms_sys/13(OMAPve_y_ADAS_AEBMassageDisp) -> OMAPve_y_ADAS_AEBMassageDisp/1
  Runnable_OMAP_10ms_sys/14(OMAPve_g_ADAS_ACCTorqueReq) -> OMAPve_g_ADAS_ACCTorqueReq/1
  LKASve_y_EPS_State_Control/1 -> Runnable_OMAP_10ms_sys/73(LKASve_y_EPS_State_Control)
  Runnable_OMAP_10ms_sys/46(OMAPve_y_ADAS_ESARequest) -> OMAPve_y_ADAS_ESARequest/1
  Runnable_OMAP_10ms_sys/10(OMAPve_y_ADAS_AEBAlertReq) -> OMAPve_y_ADAS_AEBAlertReq/1
  IMAPve_g_R0_C0/1 -> Runnable_OMAP_10ms_sys/109(IMAPve_g_R0_C0)
  Runnable_OMAP_10ms_sys/8(OMAPve_y_ADAS_ACC_RVVReqType) -> OMAPve_y_ADAS_ACC_RVVReqType/1
  Runnable_OMAP_10ms_sys/7(OMAPve_y_ADAS_ACCStatusIconDis) -> OMAPve_y_ADAS_ACCStatusIconDis/1
  Runnable_OMAP_10ms_sys/6(OMAPve_y_ADAS_ACCSetSpeedDis) -> OMAPve_y_ADAS_ACCSetSpeedDis/1
  Runnable_OMAP_10ms_sys/5(OMAPve_y_ADAS_ACCSetSpeed) -> OMAPve_y_ADAS_ACCSetSpeed/1
  Runnable_OMAP_10ms_sys/16(OMAPve_g_ADAS_DownorUpGearMinTime) -> OMAPve_g_ADAS_DownorUpGearMinTime/1
  Runnable_OMAP_10ms_sys/45(OMAPve_g_ADAS_ESATorqueReq) -> OMAPve_g_ADAS_ESATorqueReq/1
  ICABve_d_ICAMode/1 -> Runnable_OMAP_10ms_sys/96(ICABve_d_ICAMode)
  Runnable_OMAP_10ms_sys/3(OMAPve_y_ADAS_ACCHeadwayDisplay) -> OMAPve_y_ADAS_ACCHeadwayDisplay/1
  Runnable_OMAP_10ms_sys/17(OMAPve_y_ADAS_UpDownGearChange) -> OMAPve_y_ADAS_UpDownGearChange/1
  Runnable_OMAP_10ms_sys/2(OMAPve_y_ADAS_ISLCDriverRemind) -> OMAPve_y_ADAS_ISLCDriverRemind/1
  AEBSve_d_JABS_FltStatus/1 -> Runnable_OMAP_10ms_sys/47(AEBSve_d_JABS_FltStatus)
  ICABve_g_SteerAngleCmd/1 -> Runnable_OMAP_10ms_sys/95(ICABve_g_SteerAngleCmd)
  Runnable_OMAP_10ms_sys/4(OMAPve_y_ADAS_ACCHeadwayIcon) -> OMAPve_y_ADAS_ACCHeadwayIcon/1
  Runnable_OMAP_10ms_sys/51(OMAPve_y_ADAS_ESAFaultSt) -> OMAPve_y_ADAS_ESAFaultSt/1
  Runnable_OMAP_10ms_sys/12(OMAPve_y_ADAS_AEBSwitchStatus) -> OMAPve_y_ADAS_AEBSwitchStatus/1
  AEBSve_d_JABS_AlertReq/1 -> Runnable_OMAP_10ms_sys/48(AEBSve_d_JABS_AlertReq)
  ELKSve_y_ELK_Action_Indication/1 -> Runnable_OMAP_10ms_sys/82(ELKSve_y_ELK_Action_Indication)
  Runnable_OMAP_10ms_sys/11(OMAPve_y_ADAS_AEBFaultStatus) -> OMAPve_y_ADAS_AEBFaultStatus/1
  ELKSve_y_Hands_Off_Warning/1 -> Runnable_OMAP_10ms_sys/81(ELKSve_y_Hands_Off_Warning)
  Runnable_OMAP_10ms_sys/20(OMAPve_y_ADAS_DeclControlReq) -> OMAPve_y_ADAS_DeclControlReq/1
  Runnable_OMAP_10ms_sys/50(OMAPve_y_ADAS_HWATurnOnIdctr) -> OMAPve_y_ADAS_HWATurnOnIdctr/1
  ICABve_d_ICAState/1 -> Runnable_OMAP_10ms_sys/97(ICABve_d_ICAState)
  Runnable_OMAP_10ms_sys/9(OMAPve_y_ADAS_ACCMessagePrompt) -> OMAPve_y_ADAS_ACCMessagePrompt/1
  ACCSve_d_ACC_go_request/1 -> Runnable_OMAP_10ms_sys/18(ACCSve_d_ACC_go_request)
  Runnable_OMAP_10ms_sys/24(OMAPve_y_ADAS_DecelerationType) -> OMAPve_y_ADAS_DecelerationType/1
  Runnable_OMAP_10ms_sys/37(OMAPve_y_ADAS_ELKSts) -> OMAPve_y_ADAS_ELKSts/1
  LKASve_y_LKATorqueReq/1 -> Runnable_OMAP_10ms_sys/77(LKASve_y_LKATorqueReq)
  LKASve_g_LKATorqueReq_Value/1 -> Runnable_OMAP_10ms_sys/78(LKASve_g_LKATorqueReq_Value)
  ELKSve_g_LKATorqueReq_Value/1 -> Runnable_OMAP_10ms_sys/92(ELKSve_g_LKATorqueReq_Value)
  ELKSve_y_LKATorqueReq/1 -> Runnable_OMAP_10ms_sys/91(ELKSve_y_LKATorqueReq)
  ICABve_d_LKATorqueReq/1 -> Runnable_OMAP_10ms_sys/98(ICABve_d_LKATorqueReq)
  ICABve_g_LKATorqueReq_Value/1 -> Runnable_OMAP_10ms_sys/99(ICABve_g_LKATorqueReq_Value)
  IMAPve_d_APA_AutoPark_WorkSt/1 -> Runnable_OMAP_10ms_sys/113(IMAPve_d_APA_AutoPark_WorkSt)
  Runnable_OMAP_10ms_sys/57(OMAPve_g_ob019L_100) -> OMAPve_g_ob019L_100/1
  ACCSve_d_ACC_ISLCDriverRemind/1 -> Runnable_OMAP_10ms_sys/28(ACCSve_d_ACC_ISLCDriverRemind)
  ACCSve_d_ACC_ISLCState/1 -> Runnable_OMAP_10ms_sys/27(ACCSve_d_ACC_ISLCState)
  Runnable_OMAP_10ms_sys/58(OMAPve_y_ADAS_ELKPopupMessage) -> OMAPve_y_ADAS_ELKPopupMessage/1
  Runnable_OMAP_10ms_sys/59(OMAPve_y_ADAS_TurnLightsCommand) -> OMAPve_y_ADAS_TurnLightsCommand/1
  ESASve_y_LKAActivation/1 -> Runnable_OMAP_10ms_sys/120(ESASve_y_LKAActivation)
  ESASve_y_ESATorqueReq/1 -> Runnable_OMAP_10ms_sys/119(ESASve_y_ESATorqueReq)
  ESASve_y_ESARequest/1 -> Runnable_OMAP_10ms_sys/118(ESASve_y_ESARequest)
  ESASve_y_ESA_FaultSt/1 -> Runnable_OMAP_10ms_sys/117(ESASve_y_ESA_FaultSt)
  ESASve_y_ESA_State/1 -> Runnable_OMAP_10ms_sys/114(ESASve_y_ESA_State)
  ESASve_g_EPS_Factor_Control/1 -> Runnable_OMAP_10ms_sys/116(ESASve_g_EPS_Factor_Control)
  ESASve_g_ESA_SWA_CMD/1 -> Runnable_OMAP_10ms_sys/115(ESASve_g_ESA_SWA_CMD)
  ACCSve_d_ACCMessagePrompt/1 -> Runnable_OMAP_10ms_sys/26(ACCSve_d_ACCMessagePrompt)
